simulink subsystem "dcx_22l"  (R2020b)
settings: Solver=VariableStepAuto  StartTime=0.0  StopTime=10.0  RelTol=1e-3
values from neighbouring files (symbols this model uses):
  Kb = 1/22.09592    (= 0.0452572239581)    [constants.m]
  Km = 0.0452    [constants.m]
  ZE_DEN = [L R]    [constants.m]
  ZE_NUM = [1]    [constants.m]
  ZM_DEN = [(3.9774e-6 + J) B]    [constants.m]
  ZM_NUM = [1]    [constants.m]
settings Model: Creator=matti  LastModifiedBy=matti

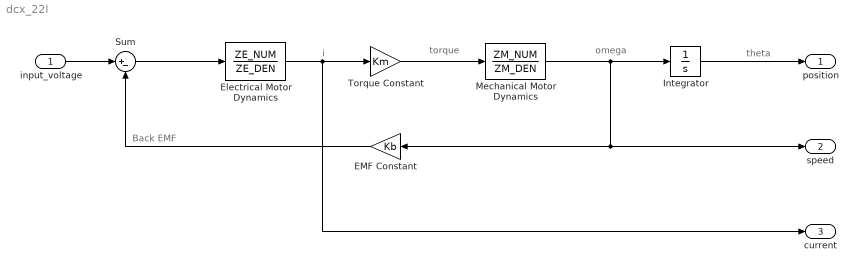
== system dcx_22l ==
  note: torque
  note: Back EMF
  note: theta
  note: i
  note: omega
  input_voltage : Inport
  EMF Constant : Gain  Gain=Kb
  Electrical Motor Dynamics : TransferFcn  Numerator=ZE_NUM  Denominator=ZE_DEN
  Integrator : Integrator
  Mechanical Motor Dynamics : TransferFcn  Numerator=ZM_NUM  Denominator=ZM_DEN
  Sum : Sum  Inputs=|+-
  Torque Constant : Gain  Gain=Km
  position : Outport
  speed : Outport  Port=2
  current : Outport  Port=3
  wires:
  input_voltage/1 -> Sum/1
  Sum/1 -> Electrical Motor Dynamics/1
  Electrical Motor Dynamics/1 -> current/1, Torque Constant/1
  EMF Constant/1 -> Sum/2
  Mechanical Motor Dynamics/1 -> speed/1, EMF Constant/1, Integrator/1
  Torque Constant/1 -> Mechanical Motor Dynamics/1
  Integrator/1 -> position/1
